simulink model "MB"  (R2016b)
settings: Solver=FixedStepDiscrete  StartTime=0.0  StopTime=inf  FixedStep=0.001  RelTol=1e-3  EnableMultiTasking=on
undefined symbols (not defined in the file or in its folder): A_Puf, B_Puf, C_Puf, infoObj, Obj
settings Model: Creator=Daniel Arbeitsplatz  LastModifiedBy=BirgerT
settings DataIOCC: LimitDataPoints=on  SaveFormat=Array  SignalLoggingSaveFormat=ModelDataLogs
settings OptimizationCC: LifeSpan=inf
settings DebuggingCC: UnderspecifiedInitializationDetection=Classic  MergeDetectMultiDrivingBlocksExec=none  SolverPrmCheckMsg=warning  MultiTaskDSMMsg=warning  MultiTaskCondExecSysMsg=none  StrictBusMsg=None  SFUnexpectedBacktrackingDiag=warning  SFNoUnconditionalDefaultTransitionDiag=warning  SFExecutionAtInitializationDiag=none
settings HardwareCC: ProdBitPerPointer=32  ProdBitPerSizeT=32  ProdBitPerPtrDiffT=32  ProdLargestAtomicFloat=None  ProdIntDivRoundTo=Undefined  ProdEndianess=Unspecified  ProdWordSize=32  ProdHWDeviceType=32-bit Generic
settings ModelReferenceCC: PropagateSignalLabelsOutOfModel=off
settings GRTTargetCC: TargetLangStandard=C89/C90 (ANSI)  GeneratePreprocessorConditionals=Disable all
settings ConfigComp: CovMetricSettings=dw  CovHtmlReporting=on  CovSaveCumulativeToWorkspaceVar=on  CovSaveSingleToWorkspaceVar=on  CovExternalEMLEnable=off  CovSFcnEnable=off

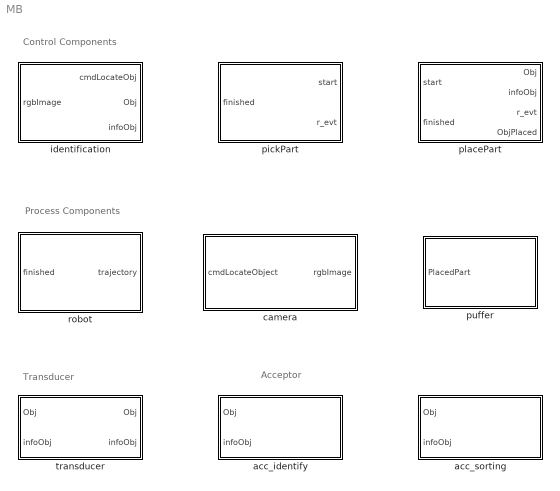
== system MB ==
  note: Acceptor
  note: Transducer
  note: Control Components
  note: Process Components
  acc_identify : Subsystem
  acc_sorting : Subsystem
  camera : Subsystem
  identification : Subsystem
  pickPart : Subsystem
  placePart : Subsystem
  puffer : Subsystem
  robot : Subsystem
  transducer : Subsystem

== system MB/acc_identify ==
  "Obj " : Inport
  infoObj : Inport  Port=2
  MATLAB Function : MATLAB Function  TreatAsAtomicUnit=on
  Stop Simulation : Stop
  wires:
  infoObj/1 -> MATLAB Function/2(infoObjIn)
  "Obj "/1 -> MATLAB Function/1(objIn)
  MATLAB Function/1(flag) -> Stop Simulation/1

== system MB/acc_sorting ==
  "Obj " : Inport
  infoObj : Inport  Port=2
  MATLAB Function : MATLAB Function  TreatAsAtomicUnit=on
  Stop Simulation : Stop
  wires:
  MATLAB Function/1(flag) -> Stop Simulation/1
  "Obj "/1 -> MATLAB Function/1(objIn)
  infoObj/1 -> MATLAB Function/2(infoObjIn)

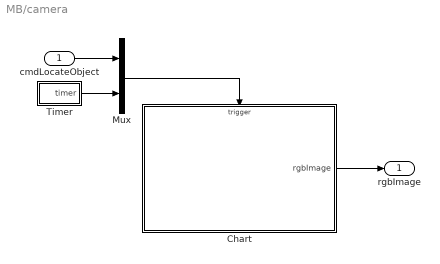
== system MB/camera ==
  cmdLocateObject : Inport
  Chart : Stateflow chart  TreatAsAtomicUnit=on
  Mux : Mux  Inputs=2
  Timer : Subsystem
  rgbImage : Outport
  wires:
  Chart/1(rgbImage) -> rgbImage/1
  Mux/1 -> Chart/Trigger
  cmdLocateObject/1 -> Mux/1
  Timer/1(timer) -> Mux/2

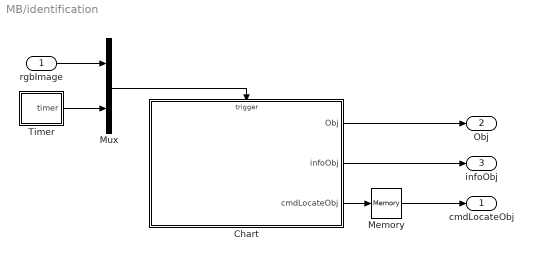
== system MB/identification ==
  rgbImage : Inport
  Chart : Stateflow chart  TreatAsAtomicUnit=on
  Memory : Memory
  Mux : Mux  Inputs=2
  Timer : Subsystem
  cmdLocateObj : Outport
  Obj : Outport  Port=2
  infoObj : Outport  Port=3
  wires:
  Chart/1(Obj) -> Obj/1
  Chart/2(infoObj) -> infoObj/1
  Mux/1 -> Chart/Trigger
  rgbImage/1 -> Mux/1
  Chart/3(cmdLocateObj) -> Memory/1
  Memory/1 -> cmdLocateObj/1
  Timer/1(timer) -> Mux/2

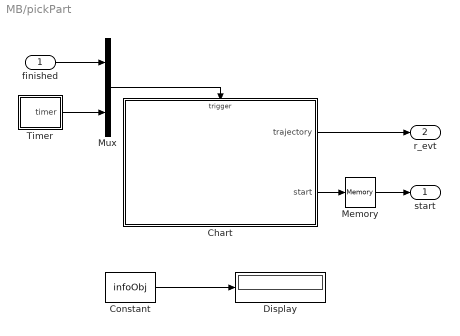
== system MB/pickPart ==
  finished : Inport
  Chart : Stateflow chart  TreatAsAtomicUnit=on
  Constant : Constant  Value=infoObj
  Display : Display
  Memory : Memory
  Mux : Mux  Inputs=2
  Timer : Subsystem
  start : Outport
  r_evt : Outport  Port=2
  wires:
  Timer/1(timer) -> Mux/2
  Memory/1 -> start/1
  Chart/2(start) -> Memory/1
  finished/1 -> Mux/1
  Mux/1 -> Chart/Trigger
  Chart/1(trajectory) -> r_evt/1
  Constant/1 -> Display/1

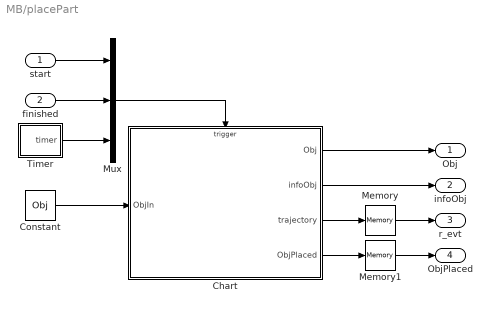
== system MB/placePart ==
  start : Inport
  finished : Inport  Port=2
  Chart : Stateflow chart  TreatAsAtomicUnit=on
  Constant : Constant  Value=Obj
  Memory : Memory
  Memory1 : Memory
  Mux : Mux  Inputs=3
  Timer : Subsystem
  Obj : Outport
  infoObj : Outport  Port=2
  r_evt : Outport  Port=3
  ObjPlaced : Outport  Port=4
  wires:
  Mux/1 -> Chart/Trigger
  start/1 -> Mux/1
  Chart/3(trajectory) -> Memory/1
  finished/1 -> Mux/2
  Memory/1 -> r_evt/1
  Chart/1(Obj) -> Obj/1
  Chart/2(infoObj) -> infoObj/1
  Chart/4(ObjPlaced) -> Memory1/1
  Memory1/1 -> ObjPlaced/1
  Constant/1 -> Chart/1(ObjIn)
  Timer/1(timer) -> Mux/3

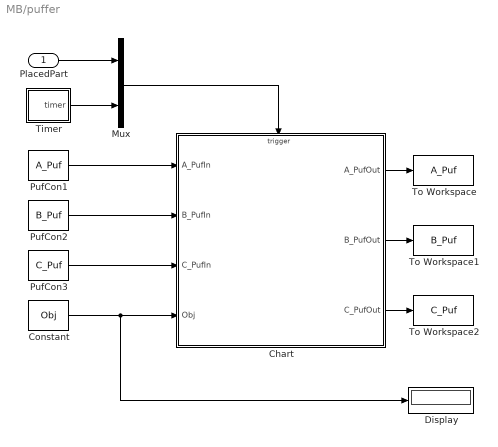
== system MB/puffer ==
  PlacedPart : Inport
  Chart : Stateflow chart  TreatAsAtomicUnit=on
  Constant : Constant  Value=Obj
  Display : Display
  Mux : Mux  Inputs=2
  PufCon1 : Constant  Value=A_Puf
  PufCon2 : Constant  Value=B_Puf
  PufCon3 : Constant  Value=C_Puf
  Timer : Subsystem
  To Workspace : ToWorkspace  VariableName=A_Puf  SampleTime=-1
      settings: MaxDataPoints=1
  To Workspace1 : ToWorkspace  VariableName=B_Puf  SampleTime=-1
      settings: MaxDataPoints=1
  To Workspace2 : ToWorkspace  VariableName=C_Puf  SampleTime=-1
      settings: MaxDataPoints=1
  wires:
  Constant/1 -> Display/1, Chart/4(Obj)
  Chart/3(C_PufOut) -> To Workspace2/1
  Chart/2(B_PufOut) -> To Workspace1/1
  Chart/1(A_PufOut) -> To Workspace/1
  PufCon3/1 -> Chart/3(C_PufIn)
  PufCon2/1 -> Chart/2(B_PufIn)
  PufCon1/1 -> Chart/1(A_PufIn)
  Mux/1 -> Chart/Trigger
  PlacedPart/1 -> Mux/1
  Timer/1(timer) -> Mux/2

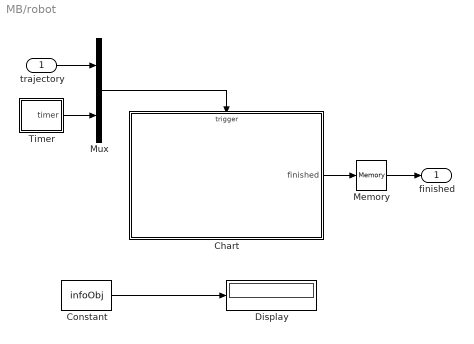
== system MB/robot ==
  trajectory : Inport
  Chart : Stateflow chart  TreatAsAtomicUnit=on
  Constant : Constant  Value=infoObj
  Display : Display
  Memory : Memory
  Mux : Mux  Inputs=2
  Timer : Subsystem
  finished : Outport
  wires:
  Mux/1 -> Chart/Trigger
  trajectory/1 -> Mux/1
  Chart/1(finished) -> Memory/1
  Memory/1 -> finished/1
  Timer/1(timer) -> Mux/2
  Constant/1 -> Display/1

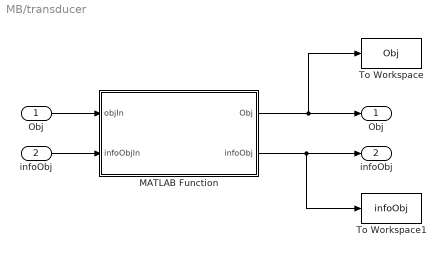
== system MB/transducer ==
  "Obj " : Inport
  infoObj : Inport  Port=2
  MATLAB Function : MATLAB Function  TreatAsAtomicUnit=on
  To Workspace : ToWorkspace  VariableName=Obj  SampleTime=-1
      settings: MaxDataPoints=1
  To Workspace1 : ToWorkspace  VariableName=infoObj  SampleTime=-1
      settings: MaxDataPoints=1
  Obj : Outport
  "infoObj " : Outport  Port=2
  wires:
  infoObj/1 -> MATLAB Function/2(infoObjIn)
  MATLAB Function/1(Obj) -> To Workspace/1, Obj/1
  "Obj "/1 -> MATLAB Function/1(objIn)
  MATLAB Function/2(infoObj) -> To Workspace1/1, "infoObj "/1

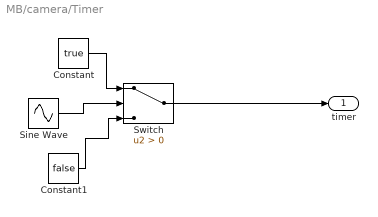
== system MB/camera/Timer ==
  Constant : Constant  Value=true
  Constant1 : Constant  Value=false
  Sine Wave : Sin  Frequency=100  SampleTime=0
  Switch : Switch  Criteria=u2 > Threshold
  timer : Outport
  wires:
  Constant1/1 -> Switch/3
  Sine Wave/1 -> Switch/2
  Constant/1 -> Switch/1
  Switch/1 -> timer/1

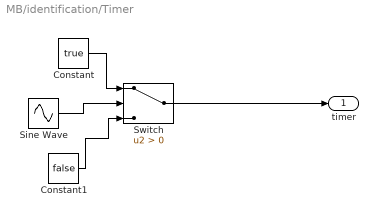
== system MB/identification/Timer ==
  Constant : Constant  Value=true
  Constant1 : Constant  Value=false
  Sine Wave : Sin  Frequency=100  SampleTime=0
  Switch : Switch  Criteria=u2 > Threshold
  timer : Outport
  wires:
  Constant1/1 -> Switch/3
  Sine Wave/1 -> Switch/2
  Constant/1 -> Switch/1
  Switch/1 -> timer/1

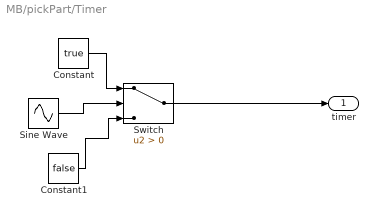
== system MB/pickPart/Timer ==
  Constant : Constant  Value=true
  Constant1 : Constant  Value=false
  Sine Wave : Sin  Frequency=100  SampleTime=0
  Switch : Switch  Criteria=u2 > Threshold
  timer : Outport
  wires:
  Switch/1 -> timer/1
  Constant/1 -> Switch/1
  Sine Wave/1 -> Switch/2
  Constant1/1 -> Switch/3

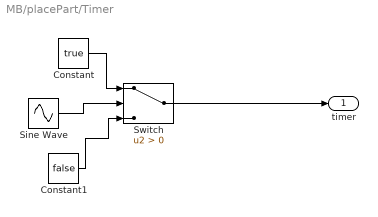
== system MB/placePart/Timer ==
  Constant : Constant  Value=true
  Constant1 : Constant  Value=false
  Sine Wave : Sin  Frequency=100  SampleTime=0
  Switch : Switch  Criteria=u2 > Threshold
  timer : Outport
  wires:
  Constant1/1 -> Switch/3
  Sine Wave/1 -> Switch/2
  Constant/1 -> Switch/1
  Switch/1 -> timer/1

== system MB/puffer/Timer ==
  Constant : Constant  Value=true
  Constant1 : Constant  Value=false
  Sine Wave : Sin  Frequency=100  SampleTime=0
  Switch : Switch  Criteria=u2 > Threshold
  timer : Outport
  wires:
  Constant1/1 -> Switch/3
  Sine Wave/1 -> Switch/2
  Constant/1 -> Switch/1
  Switch/1 -> timer/1

== system MB/robot/Timer ==
  Constant : Constant  Value=true
  Constant1 : Constant  Value=false
  Sine Wave : Sin  Frequency=100  SampleTime=0
  Switch : Switch  Criteria=u2 > Threshold
  timer : Outport
  wires:
  Constant1/1 -> Switch/3
  Sine Wave/1 -> Switch/2
  Constant/1 -> Switch/1
  Switch/1 -> timer/1

== stateflow chart MB/identification/Chart ==
  state idle
  state locatePart
    en: ml.fprintf('CM.identification send cmdLocateObj to PM.camera\n')
  state identifyObject
    ex: Obj = ml.ceil(ml.rand(1)*3);
    ml.fprintf('CM.identification: Obj= %d\n',Obj)
  note: simplified object identification
      | by random part type definition
      | (possible types are 1, 2 or 3)
  state identifyPosition
    en: infoObj = Obj;
    ml.fprintf('CM.identification: infoObj= %d\n',Obj)
  note: simplified
  (default) -> idle
  identifyPosition -> idle
  idle -> locatePart : /cmdLocateObj;
  locatePart -> identifyObject : rgbImage
  identifyObject -> identifyPosition
  data: Obj output int8 =0; infoObj output int8
  events: rgbImage input EITHER_EDGE_EVENT; cmdLocateObj output EITHER_EDGE_EVENT; time input EITHER_EDGE_EVENT

== stateflow chart MB/camera/Chart ==
  state idle
  state lookForObject
    ex: ml.disp('PM.camera send rgbImage to CM.identification')
  (default) -> idle
  lookForObject -> idle : after(1,time)/rgbImage;
  idle -> lookForObject : cmdLocateObj
  events: cmdLocateObj input EITHER_EDGE_EVENT; rgbImage output EITHER_EDGE_EVENT; time input EITHER_EDGE_EVENT

== matlab function MB/transducer/MATLAB Function ==
  data: objIn input; Obj output; infoObjIn input; infoObj output
function [Obj,infoObj] = Transducer(objIn, infoObjIn)
%Transducer
%transfers and writes values to workspace only 
%perhaps it should also write A_Puf etc to WS

Obj = objIn;
infoObj = infoObjIn;
% A_Puf = A_PufIn;
% B_Puf = B_PufIn;
% C_Puf = C_PufIn;
% switch Obj
%     case 1
%         A_Puf = A_PufIn+1;
%     case 2
%         B_Puf = B_PufIn+1;
%     case 3
%         C_Puf = C_PufIn+1;
% end

end %function

== matlab function MB/acc_identify/MATLAB Function ==
  data: objIn input; flag output; infoObjIn input
function flag = AcceptorITask(objIn, infoObjIn)
%#codegen

%AcceptorITask determines if current identification task is finished


if objIn == 0
    flag = false;
else
    flag = true;
    disp('EF.transducer saved results in SES variables')
    disp('EF.acc_identify STOPPED current SM')
end

end

== stateflow chart MB/pickPart/Chart ==
  state idle
    ex: ml.fprintf('CM.pickPart send trajectory_go to PM.robot\n')
  state approach
    ex: ml.fprintf('CM.pickPart received finished from PM.robot\n');
    ml.fprintf('CM.pickPart send trajectory_pick to PM.robot\n');
  state picking
  state depart
  state finished
    en: ml.fprintf('CM.pickPart received finished from PM.robot\n');
    ml.fprintf('CM.pickPart send start to CM.placePart\n');
  (default) -> idle
  idle -> approach : /trajectory;
  approach -> picking : finished/trajectory;
  picking -> depart : finished/trajectory;
  depart -> finished : finished/start;
  events: time input EITHER_EDGE_EVENT; trajectory output EITHER_EDGE_EVENT; finished input EITHER_EDGE_EVENT; start output EITHER_EDGE_EVENT

== stateflow chart MB/placePart/Chart ==
  state idle
    en:Obj = ObjIn;
  state approach
    en: ml.fprintf('CM.placePart received start\n');
    ml.fprintf('CM.placePart send trajectory_go to PM.robot\n');
  state placing
    en: ml.fprintf('CM.placePart received finish from PM.robot\n');
    ml.fprintf('CM.placePart send trajectory_place to PM.robot\n');
  state placed
    ex: ml.fprintf('CM.placePart received finished (PLACING) from PM.robot\n');
    ml.fprintf('CM.placePart send trajectory_goHome to PM.robot\n');
  state depart
    en: Obj = 0;
    infoObj = 0;
  (default) -> idle
  idle -> approach : start/trajectory;
  approach -> placing : finished/trajectory;
  placing -> (junction 33) : /ObjPlaced;
  (junction 33) -> placed
  placed -> depart : finished/trajectory;
  data: Obj output double =4; infoObj output double =4; ObjIn input double
  events: start input EITHER_EDGE_EVENT; trajectory output EITHER_EDGE_EVENT; finished input EITHER_EDGE_EVENT; time input EITHER_EDGE_EVENT; ObjPlaced output EITHER_EDGE_EVENT

== stateflow chart MB/robot/Chart ==
  state idle
  state move
    en:loc = ml.round(ml.rand(1)*20)+10;
  (default) -> idle
  idle -> move [order 2] : trajectoryPlace
  move -> idle : after(loc,time)/finished;
  idle -> move [order 1] : trajectoryPick
  data: loc local double =20
  events: trajectoryPick input EITHER_EDGE_EVENT; trajectoryPlace input EITHER_EDGE_EVENT; time input EITHER_EDGE_EVENT; finished output EITHER_EDGE_EVENT

== matlab function MB/acc_sorting/MATLAB Function ==
  data: objIn input; flag output; infoObjIn input
function flag = AcceptorSTask(objIn, infoObjIn)
%#codegen

%AcceptorSTask determines if current sorting task is finished 


if objIn == 0
    flag = true;
    disp('EF.transducer saved results in SES variables')
    disp('EF.acc_identify STOPPED current SM')
else
    flag = false;
end

end

== stateflow chart MB/puffer/Chart ==
  state waitForPart
  (default) -> waitForPart
  (junction 9) -> waitForPart
  waitForPart -> (junction 5) : PartPlaced
  (junction 5) -> (junction 7) [order 1] : [Obj==1]
  (junction 5) -> (junction 6) [order 2]
  (junction 7) -> (junction 12) : {A_PufOut=A_PufIn+1;}
  (junction 6) -> (junction 11) [order 1] : [Obj==2]
  (junction 6) -> (junction 13) [order 2]
  (junction 11) -> (junction 8) : {B_PufOut=B_PufIn+1;}
  (junction 13) -> (junction 14) [order 1] : [Obj==3]
  (junction 13) -> (junction 9) [order 2]
  (junction 14) -> (junction 15) : {C_PufOut=C_PufIn+1;}
  (junction 15) -> (junction 9)
  (junction 8) -> (junction 15)
  (junction 12) -> (junction 8)
  data: A_PufIn input; A_PufOut output =A_Puf; B_PufIn input; B_PufOut output =B_Puf; C_PufIn input; C_PufOut output =C_Puf; Obj input
  events: PartPlaced input EITHER_EDGE_EVENT; time input EITHER_EDGE_EVENT
